simulink model "INAIL_ROVER"  (R2025b)
settings: Solver=ode45  StartTime=0.0  StopTime=50  RelTol=1e-10
undefined symbols (not defined in the file or in its folder): alpha, L, offset, R, W, x_0
libraries: simulink x2, slpidlib x2
settings Model: Creator=mcfdo  LastModifiedBy=ema
settings SolverCC: ShapePreserveControl=EnableAll
settings ModelReferenceCC: EnableRefExpFcnMdlSchedulingChecks=on
settings RTWCC: GPUComputeCapability=3.5

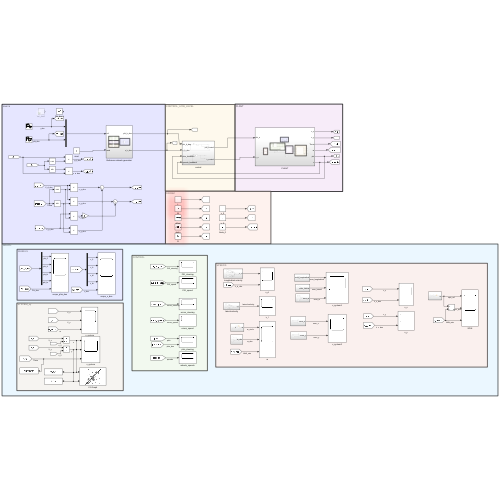
[thumbnail: Simulink's stored preview of the top-level diagram]
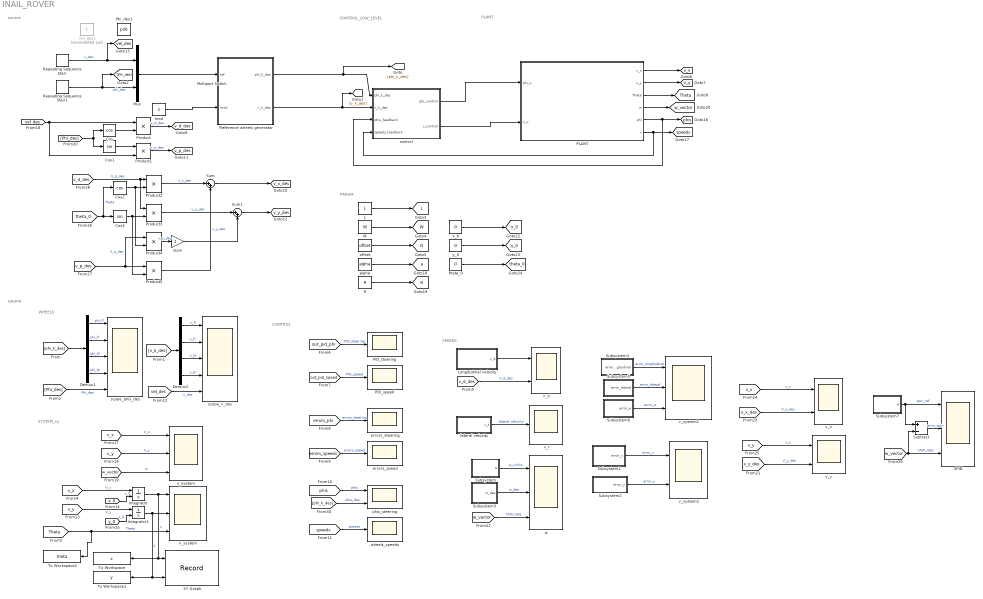
== system INAIL_ROVER ==
  note: CONTROL_LOW_LEVEL
  note: SPEEDS
  note: CONTROL
  note: SYSTEM_xy
  note: WHEELS
  note: PARAM
  note: GRAPH
  note: PLANT
  note: source
  Cos : Trigonometry  Operator=cos
  Cos1 : Trigonometry
  Cos2 : Trigonometry  Operator=cos
  Cos3 : Trigonometry
  Demux1 : Demux
  Demux2 : Demux
  Gain : Gain
  Integrator : Integrator  InitialConditionSource=external  InitialCondition=x_0
  Integrator1 : Integrator  InitialConditionSource=external  InitialCondition=x_0
  L : Constant  Value=L
  Longitudinal velocity : Subsystem
  Multiport Switch : MultiPortSwitch  SaturateOnIntegerOverflow=off  InputSameDT=off
  Mux : Mux  Inputs=2
  PID_speed : Scope
      settings: ActiveDisplayYMinimum=-1.31079  ActiveDisplayYMaximum=1.31079  DataLoggingVariableName=ScopeData5
  PID_steering : Scope
      settings: ActiveDisplayYMinimum=-3.06096  ActiveDisplayYMaximum=3.06096  DataLoggingVariableName=ScopeData4
  PLANT : Subsystem
  Phi_des1 : Constant  Value=pi/6
  Product{,1..5} (6 alike) : Product
  R : Constant  Value=R
  Reference wheels generator : Subsystem
  Repeating Sequence Stair : simulink/Sources/Repeating Sequence Stair  OutValues=[1 2 1 -1 0].'  tsamp=10  OutMin=[]  OutMax=[]  OutDataTypeStr=double  OutputDataTypeScalingMode=double  OutDataType=fixdt(0,8)  ConRadixGroup=Best Precision: Vector-wise  OutScaling=2^-12
  Repeating Sequence Stair1 : simulink/Sources/Repeating Sequence Stair  OutValues=[pi/6, pi/5, -pi/4, pi/-5, 0].'  tsamp=10  OutMin=[]  OutMax=[]  OutDataTypeStr=double  OutputDataTypeScalingMode=double  OutDataType=fixdt(0,8)  ConRadixGroup=Best Precision: Vector-wise  OutScaling=2^-12
  SPIN : Scope  NumInputPorts=3
      settings: ActiveDisplayYMinimum=-1.84564  ActiveDisplayYMaximum=0.26048  DataLoggingVariableName=ScopeData4
  Subsystem : Subsystem
  Subsystem1 : Subsystem
  Subsystem2 : Subsystem
  Subsystem3 : Subsystem
  Subsystem4 : Subsystem
  Subsystem5 : Subsystem
  Subsystem6 : Subsystem
  Subsystem7 : Subsystem
  Subtract : Sum  Inputs=+-
  Sum : Sum  Inputs=|++
  Sum1 : Sum  Inputs=|++
  To Workspace : ToWorkspace  VariableName=x  SaveFormat=Timeseries  SampleTime=-1
  To Workspace1 : ToWorkspace  VariableName=y  SaveFormat=Timeseries  SampleTime=-1
  To Workspace2 : ToWorkspace  VariableName=theta  SaveFormat=Timeseries  SampleTime=-1
  Vel_des1 : Constant  Commented=on
  W : Constant  Value=W
  XY Graph : Record  NumPorts=2.0  FileSettingsInternal="{\"entries\":[{\"content\":{\"excelSettings\":{\"content\":{},\"type\":\"Streamout.ExcelSettings\"},\"parquetSettings\":{\"content\":{},\"type\":\"Streamout.ParquetSettings\"}},\"type\":\"Streamout.FileSettingStorage\",\"uuid\":\"\"}],\"packageUris\":[\"http:\\/\\/schema.mathworks.com\\/mf0\\/streamout_blocks\\/R2020a\"],\"version\":\"1.0\"}"  FrameSettings=[0, 0]  Layout=[1 1]  SignalsInternal="{\"entries\":[{\"content\":{\"signals\":[{\"content\":{\"blockPath\":[],\"dimensions\":[1],\"domain\":\"\",\"lineColor\":\"#fe330a\",\"plots\":[ 1 ],\"port\":1,\"signalID\":1,\"signalName\":\"x\"},\"type\":\"RecordBlkView.Signal\",\"uuid\":\"\"},{\"content\":{\"blockPath\":[],\"dimensions\":[1],\"domain\":\"\",\"lineColor\":\"#22b573\",\"plots\":[ 1 ],\"port\":2,\"signalID\":2,\"signalName\":\"y\"},\"type\":\"RecordBlkView.Signal\",\"uuid\":\"\"}]},\"type\":\"RecordBlkView.InputSignals\",\"uuid\":\"\"}],\"packageUris\":[\"http:\\/\\/schema.mathworks.com\\/mf0\\/streamout_blocks\\/R2020a\"],\"version\":\"1.0\"}"  VisualizationBindings="{\"xyplotplugin\":{\"info\":[{\"series\":[{\"bindingParametersList\":[{\"parameter\":\"X-Axis\",\"signalID\":1,\"signalName\":\"x\"},{\"parameter\":\"Y-Axis\",\"signalID\":2,\"signalName\":\"y\"}],\"seriesID\":0}],\"subplotID\":1}]}}"  CompatibilityTag=XY
  alpha : Constant  Value=alpha
  control : Subsystem
  errors_speed : Scope
      settings: ActiveDisplayYMinimum=-7.08497  ActiveDisplayYMaximum=2.2646  DataLoggingVariableName=ScopeData6
  errors_steering : Scope
      settings: ActiveDisplayYMinimum=-2.12666  ActiveDisplayYMaximum=1.86874  DataLoggingVariableName=ScopeData7
  lateral velocity : Subsystem
  mod : Constant
  offset : Constant  Value=offset
  phis_steering : Scope  NumInputPorts=2
      settings: ActiveDisplayYMinimum=-1.86108  ActiveDisplayYMaximum=1.86108  DataLoggingVariableName=ScopeData9
  scope_phis_des : Scope  NumInputPorts=5
      settings: ActiveDisplayYMinimum=-2.53828  ActiveDisplayYMaximum=2.53828
  scope_v_des : Scope  NumInputPorts=5
      settings: ActiveDisplayYMinimum=0.9748  ActiveDisplayYMaximum=1.22683  DataLoggingVariableName=ScopeData2
  theta_0 : Constant  Value=0
  v_d : Scope  NumInputPorts=2
      settings: ActiveDisplayYMinimum=-0.80051  ActiveDisplayYMaximum=1.65446  DataLoggingVariableName=ScopeData3
  v_l : Scope
      settings: ActiveDisplayYMinimum=-4.2E-16  ActiveDisplayYMaximum=4.2E-16  DataLoggingVariableName=ScopeData14
  v_system : Scope  NumInputPorts=3
      settings: ActiveDisplayYMinimum=-0.17152  ActiveDisplayYMaximum=0.15258  DataLoggingVariableName=ScopeData12
  v_system1 : Scope  NumInputPorts=3
      settings: ActiveDisplayYMinimum=-1.3E-9  ActiveDisplayYMaximum=1.2E-9  DataLoggingVariableName=ScopeData13
  v_system2 : Scope  NumInputPorts=2
      settings: ActiveDisplayYMinimum=-1.01673  ActiveDisplayYMaximum=0.18916  DataLoggingVariableName=ScopeData3
  v_x : Scope  NumInputPorts=2
      settings: ActiveDisplayYMinimum=-0.11063  ActiveDisplayYMaximum=0.9957
  v_y : Scope  NumInputPorts=2
      settings: ActiveDisplayYMinimum=-0.06638  ActiveDisplayYMaximum=0.59746  DataLoggingVariableName=ScopeData2
  w : Scope  NumInputPorts=3
      settings: ActiveDisplayYMinimum=-4.37652  ActiveDisplayYMaximum=5.22281  DataLoggingVariableName=ScopeData11
  wheels_speeds : Scope
      settings: ActiveDisplayYMinimum=-0.8125  ActiveDisplayYMaximum=2.3125  DataLoggingVariableName=ScopeData8
  x_0 : Constant  Value=0
  x_system : Scope  NumInputPorts=3
      settings: ActiveDisplayYMinimum=-4.37568  ActiveDisplayYMaximum=9.5596
  y_0 : Constant  Value=0
  tag scope: L=global, O=global, R=global, Theta=global, W=global, a=global, phis=global, speeds=global, theta_0=global, v_d_des=global, v_p_des=global, v_x=global, v_x_des=global, v_y=global, v_y_des=global, vel_des=global, w_vector=global, x_0=global, y_0=global
  wires:
  Repeating Sequence Stair/1 -> [vel_des], Mux/1  "v_des"
  Repeating Sequence Stair1/1 -> [Phi_des], Mux/2  "phi_des"
  Cos/1 -> Product/2
  Product/1 -> [v_d_des]  "v_d_des"
  PLANT/5(phi) -> control/3(phis_feedback), [phis]
  PLANT/6(v) -> control/4(speeds_feedback), [speeds]
  Demux1/1 -> scope_phis_des/1  "phi_fl"
  Demux1/2 -> scope_phis_des/2  "phi_fr"
  Demux1/3 -> scope_phis_des/3  "phi_bl"
  Demux1/4 -> scope_phis_des/4  "phi_br"
  [phi_k_des] -> Demux1/1
  [v_k_des] -> Demux2/1
  Demux2/1 -> scope_v_des/1  "v_fi"
  Demux2/2 -> scope_v_des/2  "v_fr"
  Demux2/3 -> scope_v_des/3  "v_bl"
  Demux2/4 -> scope_v_des/4  "v_br"
  [Phi_des] -> scope_phis_des/5  "Phi_des"
  L/1 -> [L]
  W/1 -> [W]
  offset/1 -> [O]
  PLANT/1(v_x) -> [v_x]
  PLANT/2(v_y) -> [v_y]
  PLANT/3(Theta) -> [Theta]
  [v_d_des] -> v_d/2  "V_d_des"
  [out_pid_phi] -> PID_steering/1  "PID_steering"
  [out_pid_speed] -> PID_speed/1  "PID_speed"
  [errors_phi] -> errors_steering/1  "errors_steering"
  [errors_speeds] -> errors_speed/1  "errors_speed"
  [speeds] -> wheels_speeds/1  "speeds"
  [phis] -> phis_steering/1  "phis"
  alpha/1 -> [a]
  R/1 -> [R]
  PLANT/4(w) -> [w_vector]
  [vel_des] -> scope_v_des/5  "v_des"
  [v_x] -> v_system/1  "V_x"
  [v_y] -> v_system/2  "V_y"
  [w_vector] -> v_system/3  "w"
  Longitudinal velocity/1(v_d) -> v_d/1
  lateral velocity/1(v_t) -> v_l/1  "lateral velocity"
  Subsystem/1(w) -> w/1  "w_circle"
  Subsystem3/1(w_des) -> w/2  "w_des"
  Subsystem4/1(error_longitudinal) -> v_system1/1  "error_longitudinal"
  Subsystem5/1(error_lateral) -> v_system1/2  "error_lateral"
  Subsystem6/1(error_w) -> v_system1/3  "error_w"
  [v_y] -> Integrator1/1  "V_y"
  [v_x] -> Integrator/1  "V_x"
  theta_0/1 -> [theta_0]
  x_0/1 -> [x_0]
  y_0/1 -> [y_0]
  [Theta] -> To Workspace2/1, x_system/3  "Theta"
  Integrator/1 -> x_system/1, To Workspace/1, XY Graph/1  "x"
  Integrator1/1 -> x_system/2, To Workspace1/1, XY Graph/2  "y"
  [x_0] -> Integrator/2  "x_0"
  [y_0] -> Integrator1/2  "x_0"
  Cos1/1 -> Product1/1
  Product1/1 -> [v_p_des]  "v_p_des"
  [vel_des] -> Product/1, Product1/2
  [Phi_des] -> Cos1/1, Cos/1
  [w_vector] -> w/3  "YAW_rate"
  control/2(v_control) -> PLANT/2(v_u)
  control/1(phi_control) -> PLANT/1(phi_u)
  Reference wheels generator/1(phi_k_des) -> [phi_k_des], control/1(phi_k_des)
  Reference wheels generator/2(v_k_des) -> [v_k_des], control/2(v_k_des)
  Mux/1 -> Reference wheels generator/1(ref)
  mod/1 -> Reference wheels generator/2(mod)
  [v_x_des] -> v_x/2  "V_x_des"
  [v_x] -> v_x/1  "v_x"
  [v_y] -> v_y/1  "v_y"
  [v_y_des] -> v_y/2  "V_y_des"
  Subsystem1/1(error_x) -> v_system2/1  "error_x"
  Subsystem2/1(error_y) -> v_system2/2  "error_y"
  Cos2/1 -> Product2/2, Product4/2
  Cos3/1 -> Product3/2, Product5/2
  [theta_0] -> Cos2/1, Cos3/1  "Theta"
  [v_d_des] -> Product3/1, Product2/1  "V_d_des"
  [v_p_des] -> Product4/1, Product5/1  "V_p_des"
  Product4/1 -> Gain/1  "v_y_des"
  Product2/1 -> Sum/1  "v_x_des"
  Sum/1 -> [v_x_des]
  Product3/1 -> Sum1/1  "v_y_des"
  Sum1/1 -> [v_y_des]
  Gain/1 -> Sum1/2
  Product5/1 -> Sum/2  "v_y_des"
  [w_vector] -> Subtract/2, SPIN/3  "YAW_rate"
  Subsystem7/1(w) -> SPIN/1, Subtract/1  "spin_ref"
  Subtract/1 -> SPIN/2  "error_spin"
  [phi_k_des] -> phis_steering/2  "phis_des"

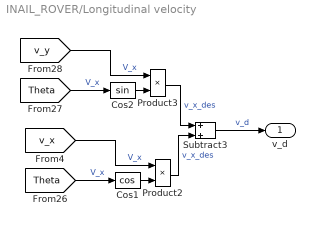
== system INAIL_ROVER/Longitudinal velocity ==
  Cos1 : Trigonometry  Operator=cos
  Cos2 : Trigonometry
  Product2 : Product
  Product3 : Product
  Subtract3 : Sum
  v_d : Outport
  wires:
  Cos2/1 -> Product3/2
  [v_x] -> Product2/1  "V_x"
  [Theta] -> Cos1/1  "V_x"
  [Theta] -> Cos2/1  "V_x"
  Product2/1 -> Subtract3/2  "v_x_des"
  [v_y] -> Product3/1  "V_x"
  Product3/1 -> Subtract3/1  "v_x_des"
  Cos1/1 -> Product2/2
  Subtract3/1 -> v_d/1  "v_d"

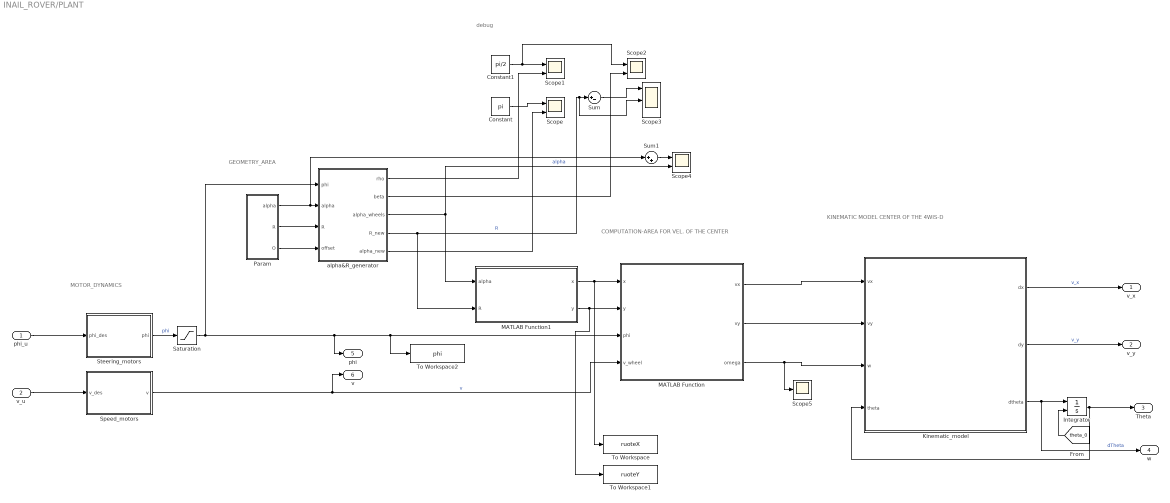
== system INAIL_ROVER/PLANT ==
  note: KINEMATIC MODEL CENTER OF THE 4WIS-D
  note: COMPUTATION-AREA FOR VEL. OF THE CENTER
  note: GEOMETRY_AREA
  note: MOTOR_DYNAMICS
  note: debug
  phi_u : Inport
  v_u : Inport  Port=2
  Constant : Constant  Value=pi
  Constant1 : Constant  Value=pi/2
  Integrator : Integrator  InitialConditionSource=external
  Kinematic_model : MATLAB Function  TreatAsAtomicUnit=on
  MATLAB Function : MATLAB Function  TreatAsAtomicUnit=on
  MATLAB Function1 : MATLAB Function  TreatAsAtomicUnit=on
  Param : Subsystem
  Saturation : Saturate  UpperLimit=pi/3  LowerLimit=-pi/3
  Scope{,1..2,4} (4 alike) : Scope  NumInputPorts=2
      Scope settings: ActiveDisplayYMinimum=0.17643  ActiveDisplayYMaximum=3.47105
      Scope1 settings: ActiveDisplayYMinimum=-0.19635  ActiveDisplayYMaximum=1.76715
      Scope2 settings: ActiveDisplayYMinimum=1.36367  ActiveDisplayYMaximum=3.43491  DataLoggingVariableName=ScopeData2
      Scope4 settings: ActiveDisplayYMinimum=-0.21061  ActiveDisplayYMaximum=6.49379  DataLoggingVariableName=ScopeData6
  Scope3 : Scope  NumInputPorts=3
      settings: ActiveDisplayYMinimum=0.56835  ActiveDisplayYMaximum=0.64277  DataLoggingVariableName=ScopeData5
  Scope5 : Scope
      settings: ActiveDisplayYMinimum=-0.21266  ActiveDisplayYMaximum=1.91394  DataLoggingVariableName=ScopeData7
  Speed_motors : Subsystem
  Steering_motors : Subsystem
  Sum : Sum  Inputs=|+-
  Sum1 : Sum  Inputs=|++
  To Workspace : ToWorkspace  VariableName=ruoteX  SaveFormat=Timeseries  SampleTime=-1
  To Workspace1 : ToWorkspace  VariableName=ruoteY  SaveFormat=Timeseries  SampleTime=-1
  To Workspace2 : ToWorkspace  VariableName=phi  SaveFormat=Timeseries  SampleTime=-1
  alpha&R_generator : MATLAB Function  TreatAsAtomicUnit=on
  v_x : Outport
  v_y : Outport  Port=2
  Theta : Outport  Port=3
  w : Outport  Port=4
  phi : Outport  Port=5
  v : Outport  Port=6
  wires:
  Steering_motors/1(phi) -> Saturation/1  "phi"
  Speed_motors/1(v) -> MATLAB Function/4(v_wheel), v/1  "v"
  Integrator/1 -> Kinematic_model/4(theta), Theta/1
  Kinematic_model/2(dy) -> v_y/1  "v_y"
  Kinematic_model/3(dtheta) -> Integrator/1, w/1  "dTheta"
  phi_u/1 -> Steering_motors/1(phi_des)
  Kinematic_model/1(dx) -> v_x/1  "v_x"
  v_u/1 -> Speed_motors/1(v_des)
  Param/1(alpha) -> Sum1/1, alpha&R_generator/2(alpha)
  Param/2(R) -> alpha&R_generator/3(R)
  Param/3(O) -> alpha&R_generator/4(offset)
  [theta_0] -> Integrator/2
  MATLAB Function1/1(x) -> To Workspace/1, MATLAB Function/1(x)
  MATLAB Function1/2(y) -> MATLAB Function/2(y), To Workspace1/1
  alpha&R_generator/4(R_new) -> Scope3/2, Sum/1, MATLAB Function1/2(R)  "R"
  alpha&R_generator/3(alpha_wheels) -> Scope4/2, MATLAB Function1/1(alpha)  "alpha"
  Constant/1 -> Scope/1
  alpha&R_generator/1(rho) -> Scope1/2
  Constant1/1 -> Scope2/1, Scope1/1
  alpha&R_generator/2(beta) -> Scope2/2
  alpha&R_generator/5(alpha_new) -> Scope/2
  MATLAB Function/1(vx) -> Kinematic_model/1(vx)
  MATLAB Function/2(vy) -> Kinematic_model/2(vy)
  MATLAB Function/3(omega) -> Scope5/1, Kinematic_model/3(w)
  Sum/1 -> Scope3/1
  Sum1/1 -> Scope4/1
  Saturation/1 -> To Workspace2/1, MATLAB Function/3(phi), phi/1, alpha&R_generator/1(phi)

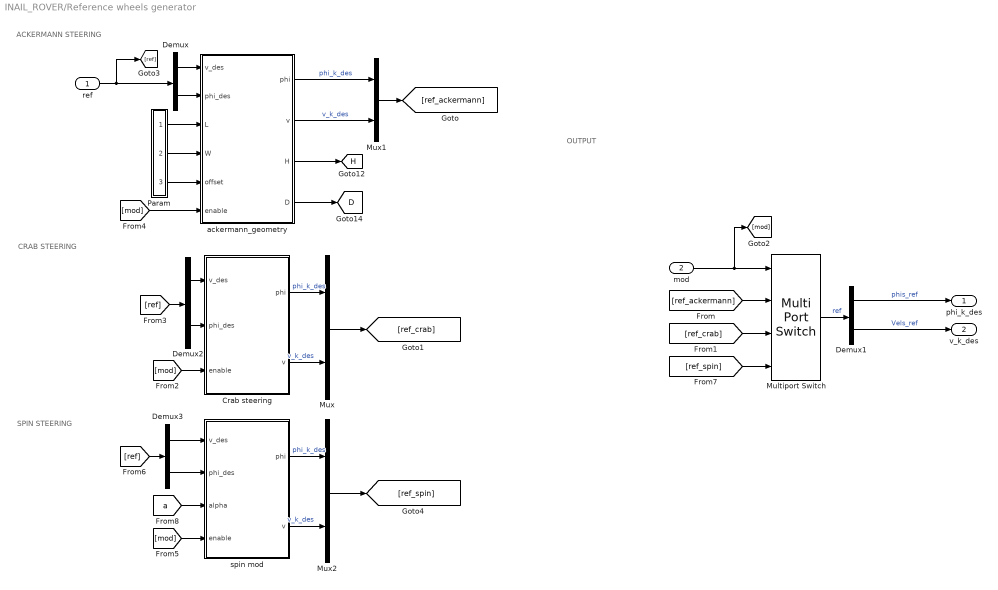
== system INAIL_ROVER/Reference wheels generator ==
  note: SPIN STEERING
  note: CRAB STEERING
  note: ACKERMANN STEERING
  note: OUTPUT
  ref : Inport
  mod : Inport  Port=2
  Crab steering : MATLAB Function  TreatAsAtomicUnit=on
  Demux{,1..3} (4 alike) : Demux  Outputs=2
  Multiport Switch : MultiPortSwitch  SaturateOnIntegerOverflow=off  InputSameDT=off
  Mux : Mux  Inputs=2
  Mux1 : Mux  Inputs=2
  Mux2 : Mux  Inputs=2
  Param : Subsystem
  ackermann_geometry : MATLAB Function  TreatAsAtomicUnit=on
  spin mod : MATLAB Function  TreatAsAtomicUnit=on
  phi_k_des : Outport
  v_k_des : Outport  Port=2
  tag scope: D=global, H=global
  wires:
  ref/1 -> [ref], Demux/1
  Param/2(W) -> ackermann_geometry/4(W)
  Demux/2 -> ackermann_geometry/2(phi_des)
  ackermann_geometry/4(D) -> [D]
  Param/1(L) -> ackermann_geometry/3(L)
  ackermann_geometry/3(H) -> [H]
  Demux/1 -> ackermann_geometry/1(v_des)
  Param/3(O) -> ackermann_geometry/5(offset)
  mod/1 -> [mod], Multiport Switch/1
  Crab steering/1(phi) -> Mux/1  "phi_k_des"
  Crab steering/2(v) -> Mux/2  "v_k_des"
  ackermann_geometry/1(phi) -> Mux1/1  "phi_k_des"
  ackermann_geometry/2(v) -> Mux1/2  "v_k_des"
  Multiport Switch/1 -> Demux1/1  "ref"
  Demux1/1 -> phi_k_des/1  "phis_ref"
  Demux1/2 -> v_k_des/1  "Vels_ref"
  Mux1/1 -> [ref_ackermann]
  [ref_ackermann] -> Multiport Switch/2
  Mux/1 -> [ref_crab]
  [ref_crab] -> Multiport Switch/3
  [mod] -> Crab steering/3(enable)
  [ref] -> Demux2/1
  Demux2/1 -> Crab steering/1(v_des)
  Demux2/2 -> Crab steering/2(phi_des)
  [mod] -> ackermann_geometry/6(enable)
  Mux2/1 -> [ref_spin]
  Demux3/2 -> spin mod/2(phi_des)
  [ref] -> Demux3/1
  spin mod/1(phi) -> Mux2/1  "phi_k_des"
  [mod] -> spin mod/4(enable)
  spin mod/2(v) -> Mux2/2  "v_k_des"
  Demux3/1 -> spin mod/1(v_des)
  [ref_spin] -> Multiport Switch/4
  [a] -> spin mod/3(alpha)

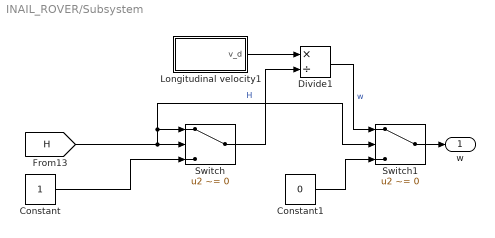
== system INAIL_ROVER/Subsystem ==
  Constant : Constant
  Constant1 : Constant  Value=0
  Divide1 : Product  Inputs=*/
  Longitudinal velocity1 : Subsystem
  Switch : Switch  Criteria=u2 ~= 0  SaturateOnIntegerOverflow=off  InputSameDT=off
  Switch1 : Switch  Criteria=u2 ~= 0  SaturateOnIntegerOverflow=off  InputSameDT=off
  w : Outport
  wires:
  Longitudinal velocity1/1(v_d) -> Divide1/1
  [H] -> Switch/1, Switch1/2, Switch/2  "H"
  Switch/1 -> Divide1/2
  Constant/1 -> Switch/3
  Divide1/1 -> Switch1/1  "w"
  Switch1/1 -> w/1
  Constant1/1 -> Switch1/3

== system INAIL_ROVER/Subsystem1 ==
  Subtract : Sum  Inputs=+-
  error_x : Outport
  wires:
  Subtract/1 -> error_x/1  "error_x"
  [v_x_des] -> Subtract/2  "V_x_des"
  [v_x] -> Subtract/1  "v_x"

== system INAIL_ROVER/Subsystem2 ==
  Subtract1 : Sum  Inputs=+-
  error_y : Outport
  wires:
  Subtract1/1 -> error_y/1  "error_y"
  [v_y] -> Subtract1/1  "v_y"
  [v_y_des] -> Subtract1/2  "V_y_des"

== system INAIL_ROVER/Subsystem3 ==
  Constant : Constant  Value=2
  Divide1 : Product  Inputs=*/
  Divide2 : Product  Inputs=*/
  w_des : Outport
  wires:
  Divide2/1 -> w_des/1  "w_des"
  [v_y_des] -> Divide2/1  "V_d_des"
  Constant/1 -> Divide1/2
  Divide1/1 -> Divide2/2  "w_des"
  [L] -> Divide1/1  "V_d_des"

== system INAIL_ROVER/Subsystem4 ==
  Longitudinal velocity1 : Subsystem
  Subtract : Sum  Inputs=+-
  error_longitudinal : Outport
  wires:
  [v_x_des] -> Subtract/2  "V_d_des"
  Longitudinal velocity1/1(v_d) -> Subtract/1  "V_x"
  Subtract/1 -> error_longitudinal/1  "error_longitudinal"

== system INAIL_ROVER/Subsystem5 ==
  Constant : Constant  Value=0
  Subtract1 : Sum  Inputs=+-
  lateral velocity1 : Subsystem
  error_lateral : Outport
  wires:
  lateral velocity1/1(v_t) -> Subtract1/1  "V_y"
  Constant/1 -> Subtract1/2  "V_y_des"
  Subtract1/1 -> error_lateral/1  "error_lateral"

== system INAIL_ROVER/Subsystem6 ==
  Subsystem2 : Subsystem
  Subsystem3 : Subsystem
  Subtract2 : Sum  Inputs=+-
  error_w : Outport
  wires:
  Subsystem2/1(w) -> Subtract2/1  "w"
  Subtract2/1 -> error_w/1  "error_w"
  Subsystem3/1(w_des) -> Subtract2/2  "w_des"

== system INAIL_ROVER/Subsystem7 ==
  Add : Sum
  Divide1 : Product  Inputs=*/
  Gain : Gain  Gain=-1
  w : Outport
  wires:
  Divide1/1 -> w/1  "spin_ref"
  [R] -> Add/1  "r"
  [O] -> Add/2  "h"
  [vel_des] -> Gain/1  "vel"
  Add/1 -> Divide1/2
  Gain/1 -> Divide1/1

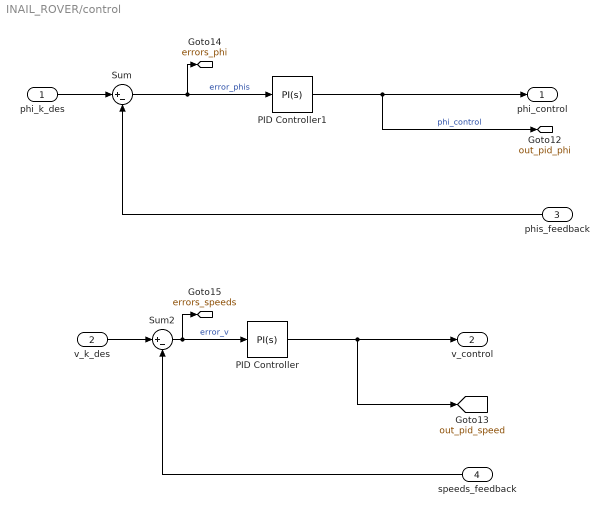
== system INAIL_ROVER/control ==
  phi_k_des : Inport
  v_k_des : Inport  Port=2
  phis_feedback : Inport  Port=3
  speeds_feedback : Inport  Port=4
  PID Controller : slpidlib/PID Controller  Controller=PI  Form=Parallel  TimeDomain=Continuous-time  UseExternalTs=off  SampleTime=-1  IntegratorMethod=Forward Euler  FilterMethod=Forward Euler  ControllerParametersSource=internal  P=3.537  I=4.185  UseKiTs=off  D=0  N=100  UseFilter=on  TunerSelectOption=Transfer Function Based (PID Tuner App)  InitialConditionSource=internal  InitialConditionForIntegrator=0  InitialConditionForFilter=0  DifferentiatorICPrevScaledInput=0  ExternalReset=none  TrackingMode=off  Kt=1  LimitOutput=off  SatLimitsSource=internal  UpperSaturationLimit=inf  LowerSaturationLimit=-inf  LinearizeAsGain=on  AntiWindupMode=none  Kb=1  POutMin=[]  POutMax=[]  IOutMin=[]  IOutMax=[]  DOutMin=[]  DOutMax=[]  NOutMin=[]  NOutMax=[]  SumOutMin=[]  SumOutMax=[]  SaturationOutMin=[]  SaturationOutMax=[]  PParamMin=[]  PParamMax=[]  IParamMin=[]  IParamMax=[]  DParamMin=[]  DParamMax=[]  NParamMin=[]  NParamMax=[]  KbParamMin=[]  KbParamMax=[]  KtParamMin=[]  KtParamMax=[]  KbOutMin=[]  KbOutMax=[]  KtOutMin=[]  KtOutMax=[]  IntegratorOutMin=[]  IntegratorOutMax=[]  FilterOutMin=[]  FilterOutMax=[]  SumI1OutMin=[]  SumI1OutMax=[]  SumI2OutMin=[]  SumI2OutMax=[]  SumI3OutMin=[]  SumI3OutMax=[]  SumI4OutMin=[]  SumI4OutMax=[]  SumDOutMin=[]  SumDOutMax=[]  DifferentiatorOutMin=[]  DifferentiatorOutMax=[]  FilterDiffOutCoefMin=[]  FilterDiffOutCoefMax=[]  ReciprocalOutMin=[]  ReciprocalOutMax=[]  SumDenOutMin=[]  SumDenOutMax=[]  SumNumOutMin=[]  SumNumOutMax=[]  DivideOutMin=[]  DivideOutMax=[]  UdiffTsProdOutMin=[]  UdiffTsProdOutMax=[]  NTsProdOutMin=[]  NTsProdOutMax=[]  UintegralTsProdOutMin=[]  UintegralTsProdOutMax=[]  UngainTsProdOutMin=[]  UngainTsProdOutMax=[]  IntegratorContinuousStateAttributes=''  IntegratorStateMustResolveToSignalObject=off  IntegratorRTWStateStorageClass=Auto  FilterContinuousStateAttributes=''  FilterStateMustResolveToSignalObject=off  FilterRTWStateStorageClass=Auto  ParallelPVariant=InternalParameters  IdealPVariant=Disabled  IVariant=InternalParameters  DVariant=Disabled  IntegratorVariant=Continuous  SatVariant=Disabled  AWVariant=Passthrough  PCopyVariant=Disabled  TRVariant=Disabled  FdbkBlocksVariant=Forward  IdealPFdbkVariant=Disabled  SatFdbkVariant=Disabled  DerivativeFilterVariant=Disabled  NVariant=Disabled  NCopyVariant=Disabled_SignalSpec  FilterICVariant=Disabled  IntegratorICVariant=InternalICs  ExternalResetVariant=Disabled  TRSumVariant=Passthrough  SumFdbkVariant=Disabled  SumVariant=Sum_PI  TsampFilterVariant=InternalTs  TsampNgainVariant=Passthrough  TsampIntegralVariant=Passthrough  ExternalSaturationOutDataTypeStr=Inherit: Same as second input  aMode=0
  PID Controller1 : slpidlib/PID Controller  Controller=PI  Form=Parallel  TimeDomain=Continuous-time  UseExternalTs=off  SampleTime=-1  IntegratorMethod=Forward Euler  FilterMethod=Forward Euler  ControllerParametersSource=internal  P=3.537  I=4.185  UseKiTs=off  D=0  N=100  UseFilter=on  TunerSelectOption=Transfer Function Based (PID Tuner App)  InitialConditionSource=internal  InitialConditionForIntegrator=0  InitialConditionForFilter=0  DifferentiatorICPrevScaledInput=0  ExternalReset=none  TrackingMode=off  Kt=1  LimitOutput=off  SatLimitsSource=internal  UpperSaturationLimit=inf  LowerSaturationLimit=-inf  LinearizeAsGain=on  AntiWindupMode=none  Kb=1  POutMin=[]  POutMax=[]  IOutMin=[]  IOutMax=[]  DOutMin=[]  DOutMax=[]  NOutMin=[]  NOutMax=[]  SumOutMin=[]  SumOutMax=[]  SaturationOutMin=[]  SaturationOutMax=[]  PParamMin=[]  PParamMax=[]  IParamMin=[]  IParamMax=[]  DParamMin=[]  DParamMax=[]  NParamMin=[]  NParamMax=[]  KbParamMin=[]  KbParamMax=[]  KtParamMin=[]  KtParamMax=[]  KbOutMin=[]  KbOutMax=[]  KtOutMin=[]  KtOutMax=[]  IntegratorOutMin=[]  IntegratorOutMax=[]  FilterOutMin=[]  FilterOutMax=[]  SumI1OutMin=[]  SumI1OutMax=[]  SumI2OutMin=[]  SumI2OutMax=[]  SumI3OutMin=[]  SumI3OutMax=[]  SumI4OutMin=[]  SumI4OutMax=[]  SumDOutMin=[]  SumDOutMax=[]  DifferentiatorOutMin=[]  DifferentiatorOutMax=[]  FilterDiffOutCoefMin=[]  FilterDiffOutCoefMax=[]  ReciprocalOutMin=[]  ReciprocalOutMax=[]  SumDenOutMin=[]  SumDenOutMax=[]  SumNumOutMin=[]  SumNumOutMax=[]  DivideOutMin=[]  DivideOutMax=[]  UdiffTsProdOutMin=[]  UdiffTsProdOutMax=[]  NTsProdOutMin=[]  NTsProdOutMax=[]  UintegralTsProdOutMin=[]  UintegralTsProdOutMax=[]  UngainTsProdOutMin=[]  UngainTsProdOutMax=[]  IntegratorContinuousStateAttributes=''  IntegratorStateMustResolveToSignalObject=off  IntegratorRTWStateStorageClass=Auto  FilterContinuousStateAttributes=''  FilterStateMustResolveToSignalObject=off  FilterRTWStateStorageClass=Auto  ParallelPVariant=InternalParameters  IdealPVariant=Disabled  IVariant=InternalParameters  DVariant=Disabled  IntegratorVariant=Continuous  SatVariant=Disabled  AWVariant=Passthrough  PCopyVariant=Disabled  TRVariant=Disabled  FdbkBlocksVariant=Forward  IdealPFdbkVariant=Disabled  SatFdbkVariant=Disabled  DerivativeFilterVariant=Disabled  NVariant=Disabled  NCopyVariant=Disabled_SignalSpec  FilterICVariant=Disabled  IntegratorICVariant=InternalICs  ExternalResetVariant=Disabled  TRSumVariant=Passthrough  SumFdbkVariant=Disabled  SumVariant=Sum_PI  TsampFilterVariant=InternalTs  TsampNgainVariant=Passthrough  TsampIntegralVariant=Passthrough  ExternalSaturationOutDataTypeStr=Inherit: Same as second input  aMode=0
  Sum : Sum  Inputs=|+-
  Sum2 : Sum  Inputs=|+-
  phi_control : Outport
  v_control : Outport  Port=2
  tag scope: errors_phi=global, errors_speeds=global, out_pid_phi=global, out_pid_speed=global
  wires:
  Sum2/1 -> [errors_speeds], PID Controller/1  "error_v"
  phi_k_des/1 -> Sum/1
  speeds_feedback/1 -> Sum2/2
  PID Controller1/1 -> [out_pid_phi], phi_control/1  "phi_control"
  Sum/1 -> PID Controller1/1, [errors_phi]  "error_phis"
  phis_feedback/1 -> Sum/2
  v_k_des/1 -> Sum2/1
  PID Controller/1 -> [out_pid_speed], v_control/1

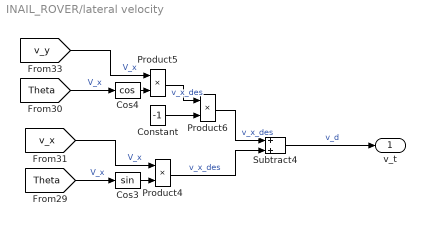
== system INAIL_ROVER/lateral velocity ==
  Constant : Constant  Value=-1
  Cos3 : Trigonometry
  Cos4 : Trigonometry  Operator=cos
  Product4 : Product
  Product5 : Product
  Product6 : Product
  Subtract4 : Sum
  v_t : Outport
  wires:
  Product5/1 -> Product6/1  "v_x_des"
  [Theta] -> Cos3/1  "V_x"
  Cos3/1 -> Product4/2
  [Theta] -> Cos4/1  "V_x"
  [v_y] -> Product5/1  "V_x"
  Cos4/1 -> Product5/2
  Product4/1 -> Subtract4/2  "v_x_des"
  [v_x] -> Product4/1  "V_x"
  Constant/1 -> Product6/2
  Product6/1 -> Subtract4/1  "v_x_des"
  Subtract4/1 -> v_t/1  "v_d"

== system INAIL_ROVER/PLANT/Param ==
  alpha : Outport
  R : Outport  Port=2
  O : Outport  Port=3
  wires:
  [a] -> alpha/1
  [R] -> R/1
  [O] -> O/1

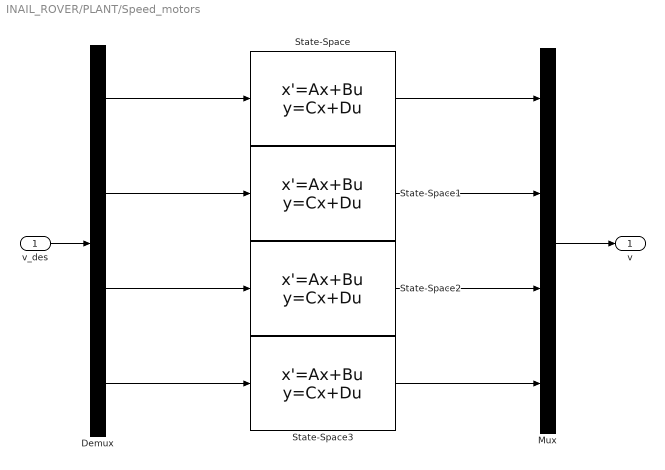
== system INAIL_ROVER/PLANT/Speed_motors ==
  v_des : Inport
  Demux : Demux
  Mux : Mux
  State-Space{,1..3} (4 alike) : StateSpace  A=[0 1; -12.25 -14]  B=[0; 12.25]  C=[1 0]  D=0  InitialCondition=0
  v : Outport
  wires:
  State-Space1/1 -> Mux/2
  State-Space2/1 -> Mux/3
  Demux/2 -> State-Space1/1
  State-Space3/1 -> Mux/4
  Demux/3 -> State-Space2/1
  Demux/4 -> State-Space3/1
  Demux/1 -> State-Space/1
  v_des/1 -> Demux/1
  State-Space/1 -> Mux/1
  Mux/1 -> v/1

== system INAIL_ROVER/PLANT/Steering_motors ==
  phi_des : Inport
  Demux : Demux
  Mux : Mux
  State-Space : StateSpace  A=[0 1; -12.25 -14]  B=[0; 12.25]  C=[1 0]  D=0  InitialCondition=[0;0 ]
  State-Space1 : StateSpace  A=[0 1; -12.25 -14]  B=[0; 12.25]  C=[1 0]  D=0  InitialCondition=0
  State-Space2 : StateSpace  A=[0 1; -12.25 -14]  B=[0; 12.25]  C=[1 0]  D=0  InitialCondition=0
  State-Space3 : StateSpace  A=[0 1; -12.25 -14]  B=[0; 12.25]  C=[1 0]  D=0  InitialCondition=0
  phi : Outport
  wires:
  State-Space1/1 -> Mux/2
  State-Space2/1 -> Mux/3
  Demux/2 -> State-Space1/1
  State-Space3/1 -> Mux/4
  Demux/3 -> State-Space2/1
  Demux/4 -> State-Space3/1
  Demux/1 -> State-Space/1
  phi_des/1 -> Demux/1
  State-Space/1 -> Mux/1
  Mux/1 -> phi/1

== system INAIL_ROVER/Reference wheels generator/Param ==
  L : Outport
  W : Outport  Port=2
  O : Outport  Port=3
  wires:
  [L] -> L/1
  [O] -> O/1
  [W] -> W/1

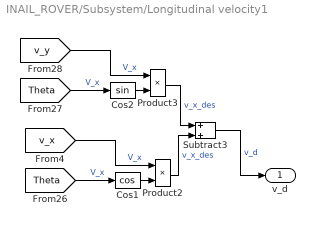
== system INAIL_ROVER/Subsystem/Longitudinal velocity1 ==
  Cos1 : Trigonometry  Operator=cos
  Cos2 : Trigonometry
  Product2 : Product
  Product3 : Product
  Subtract3 : Sum
  v_d : Outport
  wires:
  Cos2/1 -> Product3/2
  [v_x] -> Product2/1  "V_x"
  [Theta] -> Cos1/1  "V_x"
  [Theta] -> Cos2/1  "V_x"
  Product2/1 -> Subtract3/2  "v_x_des"
  [v_y] -> Product3/1  "V_x"
  Product3/1 -> Subtract3/1  "v_x_des"
  Cos1/1 -> Product2/2
  Subtract3/1 -> v_d/1  "v_d"

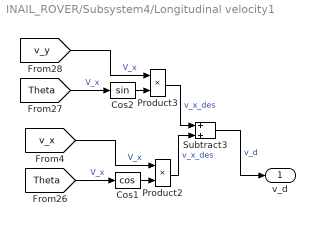
== system INAIL_ROVER/Subsystem4/Longitudinal velocity1 ==
  Cos1 : Trigonometry  Operator=cos
  Cos2 : Trigonometry
  Product2 : Product
  Product3 : Product
  Subtract3 : Sum
  v_d : Outport
  wires:
  Cos2/1 -> Product3/2
  [v_x] -> Product2/1  "V_x"
  [Theta] -> Cos1/1  "V_x"
  [Theta] -> Cos2/1  "V_x"
  Product2/1 -> Subtract3/2  "v_x_des"
  [v_y] -> Product3/1  "V_x"
  Product3/1 -> Subtract3/1  "v_x_des"
  Cos1/1 -> Product2/2
  Subtract3/1 -> v_d/1  "v_d"

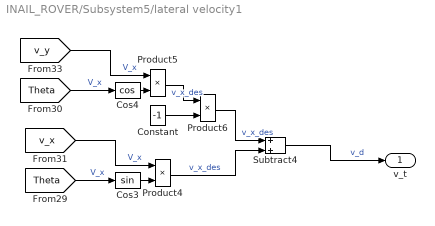
== system INAIL_ROVER/Subsystem5/lateral velocity1 ==
  Constant : Constant  Value=-1
  Cos3 : Trigonometry
  Cos4 : Trigonometry  Operator=cos
  Product4 : Product
  Product5 : Product
  Product6 : Product
  Subtract4 : Sum
  v_t : Outport
  wires:
  Product5/1 -> Product6/1  "v_x_des"
  [Theta] -> Cos3/1  "V_x"
  Cos3/1 -> Product4/2
  [Theta] -> Cos4/1  "V_x"
  [v_y] -> Product5/1  "V_x"
  Cos4/1 -> Product5/2
  Product4/1 -> Subtract4/2  "v_x_des"
  [v_x] -> Product4/1  "V_x"
  Constant/1 -> Product6/2
  Product6/1 -> Subtract4/1  "v_x_des"
  Subtract4/1 -> v_t/1  "v_d"

== system INAIL_ROVER/Subsystem6/Subsystem2 ==
  Divide1 : Product  Inputs=*/
  Longitudinal velocity1 : Subsystem
  w : Outport
  wires:
  [H] -> Divide1/2  "V_d_des"
  Divide1/1 -> w/1  "w"
  Longitudinal velocity1/1(v_d) -> Divide1/1

== system INAIL_ROVER/Subsystem6/Subsystem3 ==
  Constant : Constant  Value=2
  Divide1 : Product  Inputs=*/
  Divide2 : Product  Inputs=*/
  w_des : Outport
  wires:
  Divide2/1 -> w_des/1  "w_des"
  [v_y_des] -> Divide2/1  "V_d_des"
  Constant/1 -> Divide1/2
  Divide1/1 -> Divide2/2  "w_des"
  [L] -> Divide1/1  "V_d_des"

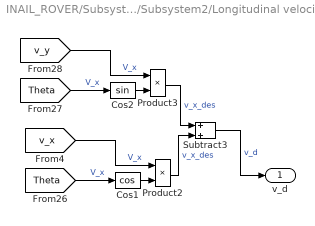
== system INAIL_ROVER/Subsystem6/Subsystem2/Longitudinal velocity1 ==
  Cos1 : Trigonometry  Operator=cos
  Cos2 : Trigonometry
  Product2 : Product
  Product3 : Product
  Subtract3 : Sum
  v_d : Outport
  wires:
  Cos2/1 -> Product3/2
  [v_x] -> Product2/1  "V_x"
  [Theta] -> Cos1/1  "V_x"
  [Theta] -> Cos2/1  "V_x"
  Product2/1 -> Subtract3/2  "v_x_des"
  [v_y] -> Product3/1  "V_x"
  Product3/1 -> Subtract3/1  "v_x_des"
  Cos1/1 -> Product2/2
  Subtract3/1 -> v_d/1  "v_d"

== matlab function INAIL_ROVER/Reference wheels generator/ackermann_geometry ==
  data: v_des input; phi_des input; phi output; v output; L input; W input; offset input; H output; D output; enable input
function [phi, v, H, D] = fcn(v_des, phi_des, L, W, offset, enable)
% fcn  calcola angoli di sterzo e velocità ruote per 4WIS secondo la
% geometria di ackerman
%
%   phi_des : direzione desiderata (rad)
%   V_des   : velocità desiderata al CG (m/s)
%   L       : passo longitudinale CG→asse anteriore (m)
%   W       : semicarreggiata (m)
%   H       : distanza CG→ICR (m)
%   offset  : distanza sterzo-ruota

phi = zeros(4,1);
v   = zeros(4,1);
H = 0;
D = L/2;
if enable ==  1
    if phi_des == 0
    
        v(1) = 1 * v_des;
        v(2) = 1 * v_des;
        v(3) = 1 * v_des;
        v(4) = 1 * v_des;
    
        phi(1) = 0;
        phi(2) = 0;
        phi(3) = 0;
        phi(4) = 0;
        H = 0;
        D = L/2;
    else
        RR = sqrt((L/2)^2 +(W/2)^2);
        H = (L/2) * cot(phi_des);%RR/cos(pi/2-0.459830833641758);%
        R = sqrt((L/2)^2 +(H)^2);
        phi_des_b = -phi_des;
        D = R;
        
        %sterzo
        phi(1) = atan2( L*sin(phi_des),   L*cos(phi_des) - W*sin(phi_des) );
        phi(2) = atan2( L*sin(phi_des),   L*cos(phi_des) + W*sin(phi_des) );
        phi(3) = atan2( L*sin(phi_des_b), L*cos(phi_des_b) + W*sin(phi_des_b) );
        phi(4) = atan2( L*sin(phi_des_b), L*cos(phi_des_b) - W*sin(phi_des_b) );
        
        
        if H >= 0
            %distanza dal ICR
            R_fl = sqrt((L/2)^2 +(H-(W/2))^2) - offset;
            R_fr = sqrt((L/2)^2 +(H+(W/2))^2) + offset;
            R_bl = sqrt((L/2)^2 +(H-(W/2))^2) - offset;
            R_br = sqrt((L/2)^2 +(H+(W/2))^2) + offset;
            
        else
            %distanza dal ICR
            R_fl = sqrt((L/2)^2 +(H-(W/2))^2) + offset;
            R_fr = sqrt((L/2)^2 +(H+(W/2))^2) - offset;
            R_bl = sqrt((L/2)^2 +(H-(W/2))^2) + offset;
            R_br = sqrt((L/2)^2 +(H+(W/2))^2) - offset;
        end
            %velocità
            v(1) = (R_fl/R) * v_des;
            v(2) = (R_fr/R) * v_des;
            v(3) = (R_bl/R) * v_des;
            v(4) = (R_br/R) * v_des;
    end
end

end

== matlab function INAIL_ROVER/PLANT/Kinematic_model ==
  data: vx input; vy input; w input; dx output; dy output; dtheta output; theta input
function [dx, dy, dtheta] = fcn(vx, vy, w, theta)
% phi(1) --- sterzo anteriore sinistro  n          |    phi(2) --- sterzo anteriore destro
% phi(3) --- sterzo posteriore sinistro            |    phi(4) --- sterzo posteriore destro
% R(1) --- distanza ruota anteriore sinistra       |    R(2) --- distanza ruota anteriore destra
% R(3) --- distanza ruota posteriore sinistra      |    R(4) --- distanza ruota posteriore destra
% v(1) --- velocita ruota anteriore sinistra       |    v(2) --- velocita ruota anteriore destra
% v(3) --- velocita ruota posteriore sinistra      |    v(4) --- velocita ruota posteriore destra
% alpha(1) --- azimut ruota anteriore sinistra     |    alpha(2) --- azimut ruota anteriore destra
% alpha(3) --- azimut ruota posteriore sinistra    |    alpha(4) --- azimut ruota posteriore destra

%dx     = (1/4) * (cos(theta + phi(1))*v(1) + cos(theta + phi(2))*v(2) + cos(theta + phi(3))*v(3) + cos(theta + phi(4))*v(4));
%dy     = (1/4) * (sin(theta + phi(1))*v(1) + sin(theta + phi(2))*v(2) + sin(theta + phi(3))*v(3) + sin(theta + phi(4))*v(4));
%dtheta = (1/4)*((1/R(1)) * sin(phi(1) - alpha(1))*v(1) + (1/R(2)) * sin(phi(2) + alpha(2))*v(2) - (1/R(3)) * sin(phi(3) + alpha(3))*v(3) - (1/R(4)) * sin(phi(4) - alpha(4))*v(4));

%W = 0.26 *2;
%L = 1.05;
%dx     = (1/4) * (cos(theta + phi(1))*v(1) + cos(theta + phi(2))*v(2) + cos(theta + phi(3))*v(3) + cos(theta + phi(4))*v(4));
%dy     = (1/4) * (sin(theta + phi(1))*v(1) + sin(theta + phi(2))*v(2) + sin(theta + phi(3))*v(3) + sin(theta + phi(4))*v(4));
%dtheta = (1/(2*sqrt(L^2+W^2)))*(sin(phi(1) - alpha)*v(1) + sin(phi(2) + alpha)*v(2) - sin(phi(3) + alpha)*v(3) - sin(phi(4) - alpha)*v(4));

    dx = vx*cos(theta) - vy*sin(theta);  % ẋ
    dy = vx*sin(theta) + vy*cos(theta);  % ẏ
    dtheta = w; 

end

== matlab function INAIL_ROVER/PLANT/alpha&R_generator ==
  data: rho output; beta output; alpha_wheels output; phi input; R_new output; alpha input; R input; offset input; alpha_new output
function [ rho, beta, alpha_wheels, R_new, alpha_new] = fcn(phi, alpha, R, offset)


R_new        = zeros(4,1);
alpha_new    = zeros(4,1);   
beta         = zeros(4,1);   
rho          = zeros(4,1);   
alpha_wheels = zeros(4,1);  

beta(1) = pi - phi(1) - (pi/2 - alpha);
beta(2) = pi + phi(2) - (pi/2 - alpha);
beta(3) = beta(1);
beta(4) = beta(2);


R_new(1) = sqrt(R^2 + offset^2 - 2*R*offset*cos(beta(1)));
R_new(2) = sqrt(R^2 + offset^2 - 2*R*offset*cos(beta(2)));
R_new(3) = sqrt(R^2 + offset^2 - 2*R*offset*cos(beta(3)));
R_new(4) = sqrt(R^2 + offset^2 - 2*R*offset*cos(beta(4)));


rho(1) = acos((R_new(1)^2 + R^2 - offset^2)/(2*R_new(1)*R));
rho(2) = acos((R_new(2)^2 + R^2 - offset^2)/(2*R_new(2)*R));
rho(3) = acos((R_new(3)^2 + R^2 - offset^2)/(2*R_new(3)*R));
rho(4) = acos((R_new(4)^2 + R^2 - offset^2)/(2*R_new(4)*R));


alpha_new(1) = alpha + rho(1);
alpha_new(2) = alpha + rho(2);
alpha_new(3) = alpha + rho(3);
alpha_new(4) = alpha + rho(4);

alpha_wheels(1) = alpha_new(1);
alpha_wheels(2) = 2*pi - alpha_new(2);
alpha_wheels(3) = pi - alpha_new(3);
alpha_wheels(4) = pi + alpha_new(4);



end

== matlab function INAIL_ROVER/PLANT/MATLAB Function ==
  data: x input; vx output; vy output; y input; phi input; v_wheel input; omega output
function [vx, vy, omega] = computeVelocityOmega(x, y, phi, v_wheel)
% computeVelocityOmega  Stima vx, vy e omega per un veicolo 4WISD
%
%   [vx, vy, omega] = computeVelocityOmega(x, y, phi, v_wheel)
%
%   Input:
%     x        : [4x1] vettore delle posizioni x delle ruote (frame veicolo)
%     y        : [4x1] vettore delle posizioni y delle ruote (frame veicolo)
%     phi      : [4x1] vettore degli angoli di sterzo [rad]
%     v_wheel  : [4x1] vettore delle velocità lineari delle ruote [m/s]
%
%   Output:
%     vx    : velocità longitudinale del veicolo [m/s]
%     vy    : velocità laterale del veicolo [m/s]
%     omega : yaw rate del veicolo [rad/s]

    % Assicura vettori colonna
    x       = x(:);
    y       = y(:);
    phi     = phi(:);
    v_wheel = v_wheel(:);

    % Matrice A (8×3) e vettore b (8×1)
    A = zeros(8,3);
    b = zeros(8,1);

    for i = 1:4
        c = cos(phi(i));
        s = sin(phi(i));

        % componente lungo l'asse della ruota
        b(2*i-1) = v_wheel(i) * c;
        b(2*i)   = v_wheel(i) * s;

        % equazioni: 
        %   vx - ω·y(i) = v_wheel·cos(phi)
        %   vy + ω·x(i) = v_wheel·sin(phi)
        A(2*i-1, :) = [1, 0, -y(i)];
        A(2*i,   :) = [0, 1,  x(i)];
    end

    % Soluzione ai minimi quadrati
    sol = (A' * A) \ (A' * b);

    vx    = sol(1);
    vy    = sol(2);
    omega = sol(3);
end

== matlab function INAIL_ROVER/PLANT/MATLAB Function1 ==
  data: alpha input; x output; R input; y output
function [x, y] = calcolaPosizioniRuote(alpha, R)
% Calcola le posizioni x e y delle 4 ruote dato R e alpha
% Input:
%   R: [4x1] vettore dei raggi (m)
%   alpha: [4x1] vettore degli angoli (rad)
% Output:
%   x: [4x1] coordinate x delle ruote
%   y: [4x1] coordinate y delle ruote

% Preallocazione
x = zeros(4,1);
y = zeros(4,1);

% Calcolo per ogni ruota
for i = 1:4
    x(i) = R(i) * cos(alpha(i));
    y(i) = R(i) * sin(alpha(i));
end

end

== matlab function INAIL_ROVER/Reference wheels generator/Crab steering ==
  data: v_des input; phi_des input; phi output; v output; enable input
function [phi, v] = fcn(v_des, phi_des, enable )
% fcn  calcola angoli di sterzo e velocità ruote per 4WIS secondo la
% geometria di ackerman
%
%   phi_des : direzione desiderata (rad)
%   V_des   : velocità desiderata al CG (m/s)
%   L       : passo longitudinale CG→asse anteriore (m)
%   W       : semicarreggiata (m)


phi = zeros(4,1);
v   = zeros(4,1);
if enable == 2
    if abs(phi_des) >= pi/3
        phi_des = pi/3;
    end
    v(1) = v_des;
    v(2) = v_des;
    v(3) = v_des;
    v(4) = v_des;

    phi(1) = phi_des;
    phi(2) = phi_des;
    phi(3) = phi_des;
    phi(4) = phi_des;

end

== matlab function INAIL_ROVER/Reference wheels generator/spin mod ==
  data: v_des input; phi_des input; alpha input; phi output; v output; enable input
function [phi, v] = fcn(v_des, phi_des, alpha, enable)
% fcn  calcola angoli di sterzo e velocità ruote per 4WIS secondo la
% geometria di ackerman
%
%   phi_des : direzione desiderata (rad)
%   V_des   : velocità desiderata al CG (m/s)
%   L       : passo longitudinale CG→asse anteriore (m)
%   W       : semicarreggiata (m)

phi = zeros(4,1);
v   = zeros(4,1);
H = 0;

if enable == 3
    v(1) = v_des;
    v(2) = -v_des;
    v(3) = v_des;
    v(4) = -v_des;

    phi(1) = -(pi/2 - alpha);
    phi(2) = pi/2 - alpha;
    phi(3) = phi(2);
    phi(4) = phi(1);

end
